simulink model "PID"  (R2017a)
settings: Solver=VariableStepAuto  StartTime=0.0  StopTime=800  FixedStep=0.01  RelTol=1e-3
undefined symbols (not defined in the file): C, R, sigbuilder_block
settings Model: Creator=Fikret Şafak  LastModifiedBy=baros

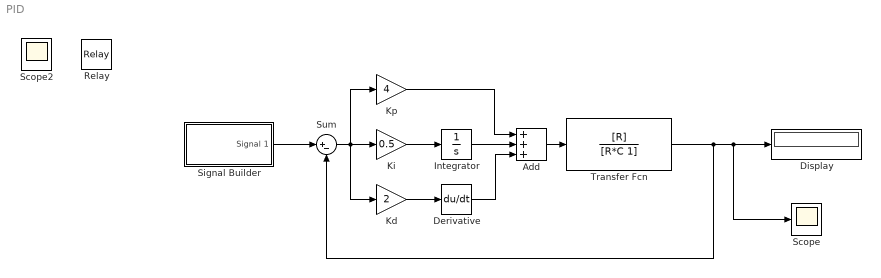
== system PID ==
  Add : Sum  Inputs=+++
  Derivative : Derivative
  Display : Display
  Integrator : Integrator
  Kd : Gain  Gain=2
  Ki : Gain  Gain=0.5
  Kp : Gain  Gain=4
  Relay : Relay  OnSwitchValue=1  OffSwitchValue=-1
  Scope : Scope
  Scope2 : Scope
  Signal Builder : Subsystem  Tag=STV Subsys  LoadFcn=sigbuilder_block('load');  StartFcn=sigbuilder_block('start');  StopFcn=sigbuilder_block('stop');  ClipboardFcn=sigbuilder_block('clipboard');  mask(Sigbuilder block){tuvar=[0:10]}
      mask help: Simulink:masks:SigbuilderBlock_MD
      mask init:
      | if ~strcmp(get_param(bdroot(gcbh),'SimulationStatus'),'stopped') tuvar = sigbuilder_block('maskInit'); end
      settings: CopyFcn=sigbuilder_block('copy');  DeleteFcn=sigbuilder_block('delete');  ModelCloseFcn=sigbuilder_block('modelClose');  PreSaveFcn=sigbuilder_block('preSave');  PauseFcn=sigbuilder_block('pause');  ContinueFcn=sigbuilder_block('continue');  NameChangeFcn=sigbuilder_block('namechange');  OpenFcn=sigbuilder_block('open',[249 129 768.6 438.6 ]);  CloseFcn=sigbuilder_block('close');
      mask Display: plot(0, 0, 100, 100,[2, 2, 32, 32, 2], [68, 8, 8, 68, 68],[32, 2], [38, 38], [32, 19, 2],[53, 60, 44], [32, 17, 17, 2],[16, 16, 31, 31]);txt = getActiveGroup(gcbh);text(2, 100, txt,'verticalAlignment', 'top');
  Sum : Sum  Inputs=|+-
  Transfer Fcn : TransferFcn  Numerator=[R]  Denominator=[R*C 1]
  wires:
  Add/1 -> Transfer Fcn/1
  Transfer Fcn/1 -> Scope/1, Display/1, Sum/2
  Sum/1 -> Kd/1, Kp/1, Ki/1
  Ki/1 -> Integrator/1
  Kd/1 -> Derivative/1
  Derivative/1 -> Add/3
  Integrator/1 -> Add/2
  Kp/1 -> Add/1
  Signal Builder/1(Signal 1) -> Sum/1

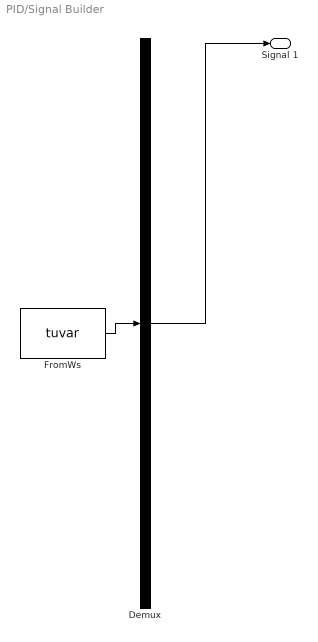
== system PID/Signal Builder ==
  Demux : Demux  Tag=STV Demux  Outputs=1
  FromWs : FromWorkspace  Tag=STV FromWs  VariableName=tuvar  SampleTime=0
      SigBuilderData=|
      | common.afterFinalStr = 'Extrapolate'
      | common.sampleTime = 0
      | dataSet.timeRange = [0 800]
      | dataSet.name = 'Group 1'
      | sbobj.Groups.Name = 'Group 1'
      | sbobj.Groups.Signals.Name = 'Signal 1'
      | sbobj.Groups.Signals.XData = [0 180 300 360 420 480 600 800]
      | sbobj.Groups.Signals.YData = [1.99842105263 2 1 1 3 3 0.5 0.5]
      | sbobj.Groups.TimeRange = [0 800]
  Signal 1 : Outport  Tag=STV Outport
  wires:
  Demux/1 -> Signal 1/1
  FromWs/1 -> Demux/1
